simulink model "es1sim"  (R2023b)
settings: Solver=VariableStepAuto  StartTime=0.0  StopTime=Tfin  RelTol=1e-3
values from neighbouring files (symbols this model uses):
  d = zeros(7,1)    [es2.m]    (also in nmpc_design_template.m)
  dv = [1e-3 1e-3 1e-3 1e-4 1e-4 1e-4 1e-3]'    [es2.m]    (also in nmpc_design_template.m)
  K = nmpc_design_st2(par)    [es2.m]    (also in nmpc_design_template.m)
  reference = [ar;eer;cir]    [es2.m]    (also in nmpc_design_template.m = [a;ee;ci])
  x0 = [r0;v0; tot_mass]    [es2.m]    (also in nmpc_design_template.m = [r0; v0; totmass])
undefined symbols (not defined in the file or in its folder): rv2oe, spacecraft_dynamics
settings Model: Creator=s331564  LastModifiedBy=luigi

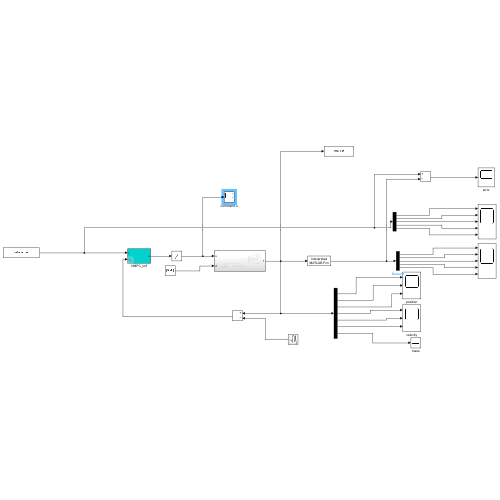
[thumbnail: Simulink's stored preview of the top-level diagram]
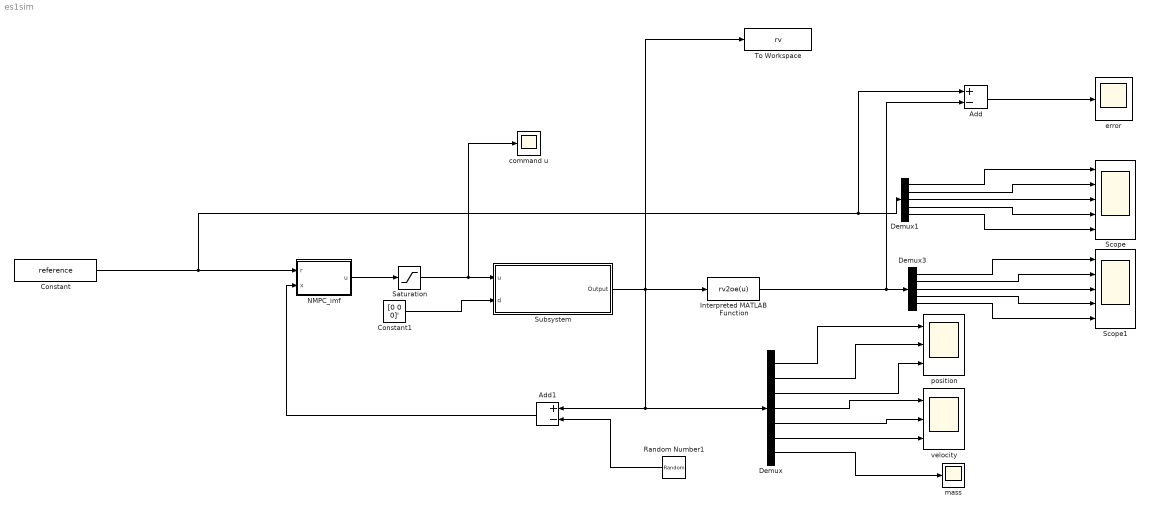
== system es1sim ==
  Add : Sum  Inputs=+-
  Add1 : Sum  Inputs=+-
  Constant : Constant  Value=reference
  Constant1 : Constant  Value=[0 0 0]'
  Demux : Demux  Outputs=7
  Demux1 : Demux  Outputs=5
  Demux3 : Demux  Outputs=5
  Interpreted MATLAB Function : MATLABFcn  MATLABFcn=rv2oe(u)
  NMPC_imf : Subsystem  mask{K=K}
      mask prompts: K "NMPC structure"
  Random Number1 : RandomNumber  Mean=d  Variance=dv  SampleTime=0.1
  Saturation : Saturate  UpperLimit=132  LowerLimit=-132
  Scope : Scope  NumInputPorts=5
  Scope1 : Scope  NumInputPorts=5
  Subsystem : Subsystem
  To Workspace : ToWorkspace  VariableName=rv  SaveFormat=Timeseries  SampleTime=-1
  command u : Scope
  error : Scope
  mass : Scope
  position : Scope  NumInputPorts=3
  velocity : Scope  NumInputPorts=3
  wires:
  Constant1/1 -> Subsystem/2(d)
  Subsystem/1(Output) -> To Workspace/1, Interpreted MATLAB Function/1, Demux/1, Add1/1
  Constant/1 -> Add/1, Demux1/1, NMPC_imf/1(r)
  Interpreted MATLAB Function/1 -> Add/2, Demux3/1
  Random Number1/1 -> Add1/2
  Add1/1 -> NMPC_imf/2(x)
  Demux/3 -> position/3
  Demux/1 -> position/1
  Demux/6 -> velocity/3
  Demux/4 -> velocity/1
  Demux/7 -> mass/1
  Demux/5 -> velocity/2
  Demux/2 -> position/2
  NMPC_imf/1(u) -> Saturation/1
  Saturation/1 -> command u/1, Subsystem/1(u)
  Add/1 -> error/1
  Demux1/1 -> Scope/1
  Demux1/2 -> Scope/2
  Demux1/3 -> Scope/3
  Demux1/4 -> Scope/4
  Demux1/5 -> Scope/5
  Demux3/5 -> Scope1/5
  Demux3/2 -> Scope1/2
  Demux3/1 -> Scope1/1
  Demux3/4 -> Scope1/4
  Demux3/3 -> Scope1/3

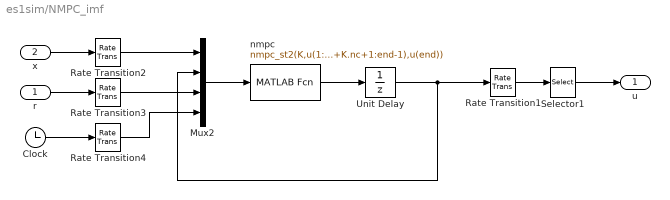
== system es1sim/NMPC_imf ==
  r : Inport
  x : Inport  Port=2
  Clock : Clock
  Mux2 : Mux
  Rate Transition{1..4} (4 alike) : RateTransition  OutPortSampleTime=K.Ts
  Selector1 : Selector  InputPortWidth=K.nc  IndexOptions=Index vector (dialog)  Indices=1:K.nu  OutputSizes=1
  Unit Delay : UnitDelay  InitialCondition=zeros(K.nc,1)  SampleTime=K.Ts  HasFrameUpgradeWarning=on
  nmpc : MATLABFcn  MATLABFcn=nmpc_st2(K,u(1:K.nx),u(K.nx+1:K.nx+K.nc),u(K.nx+K.nc+1:end-1),u(end))  OutputDimensions=K.nc
  u : Outport  PortDimensions=K.nu
  wires:
  x/1 -> Rate Transition2/1
  Unit Delay/1 -> Rate Transition1/1, Mux2/2
  Mux2/1 -> nmpc/1
  r/1 -> Rate Transition3/1
  Rate Transition2/1 -> Mux2/1
  Rate Transition1/1 -> Selector1/1
  Rate Transition3/1 -> Mux2/3
  nmpc/1 -> Unit Delay/1
  Selector1/1 -> u/1
  Clock/1 -> Rate Transition4/1
  Rate Transition4/1 -> Mux2/4

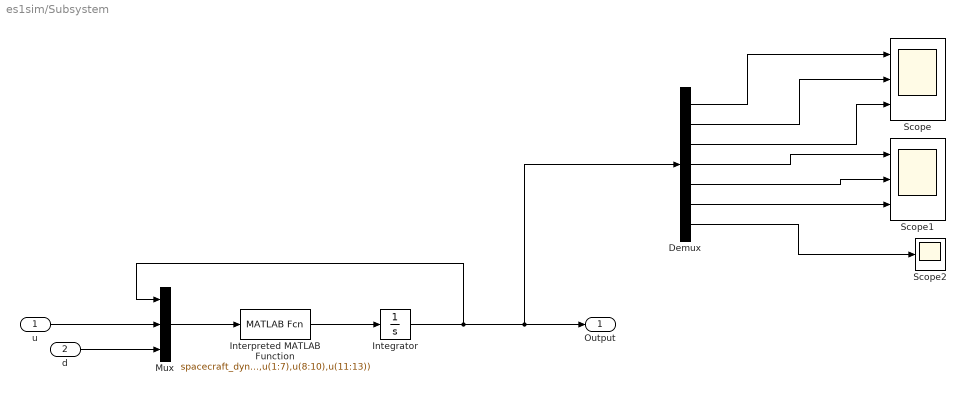
== system es1sim/Subsystem ==
  u : Inport
  d : Inport  Port=2
  Demux : Demux  Outputs=7
  Integrator : Integrator  InitialCondition=x0
  Interpreted MATLAB Function : MATLABFcn  MATLABFcn=spacecraft_dynamics(0,u(1:7),u(8:10),u(11:13))
  Mux : Mux  Inputs=3
  Scope : Scope  NumInputPorts=3
  Scope1 : Scope  NumInputPorts=3
  Scope2 : Scope
  Output : Outport
  wires:
  Demux/2 -> Scope/2
  Demux/6 -> Scope1/3
  Demux/5 -> Scope1/2
  Demux/7 -> Scope2/1
  Mux/1 -> Interpreted MATLAB Function/1
  Demux/1 -> Scope/1
  Demux/3 -> Scope/3
  Demux/4 -> Scope1/1
  Interpreted MATLAB Function/1 -> Integrator/1
  Integrator/1 -> Output/1, Demux/1, Mux/1
  u/1 -> Mux/2
  d/1 -> Mux/3
